simulink model "canPack_VCU_14"  (R2020a)
settings: Solver=VariableStepAuto  StartTime=0.0  StopTime=10.0  RelTol=1e-3
libraries: MyLibrary x1
settings Model: Creator=Administrator  LastModifiedBy=Administrator

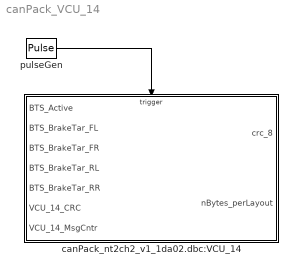
== system canPack_VCU_14 ==
  canPack_nt2ch2_v1_1da02.dbc:VCU_14 : Subsystem
  pulseGen : DiscretePulseGenerator  PulseType=Time based  Period=0.01  PulseWidth=50
  wires:
  pulseGen/1 -> canPack_nt2ch2_v1_1da02.dbc:VCU_14/Trigger

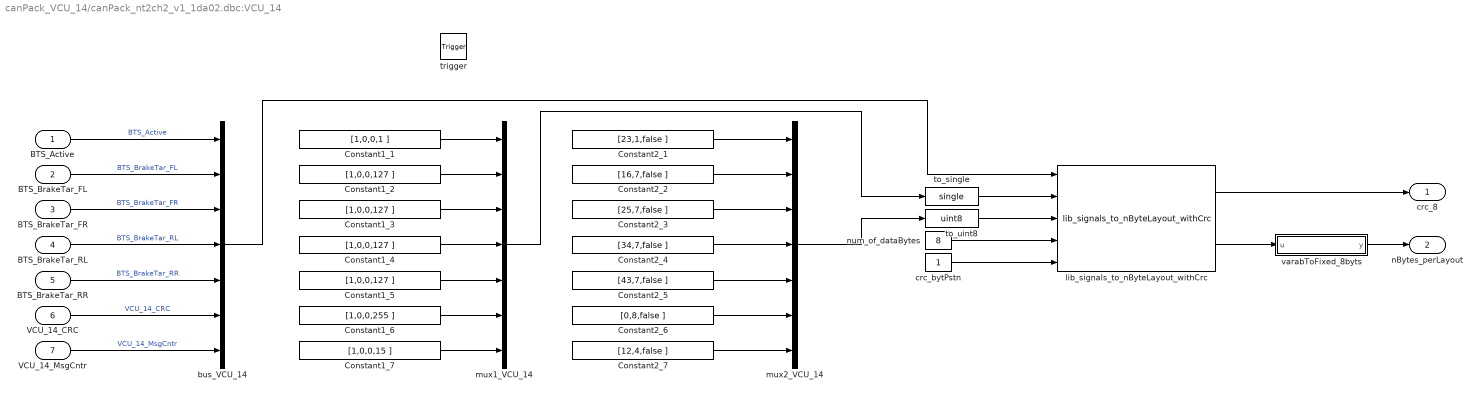
== system canPack_VCU_14/canPack_nt2ch2_v1_1da02.dbc:VCU_14 ==
  BTS_Active : Inport
  BTS_BrakeTar_FL : Inport  Port=2
  BTS_BrakeTar_FR : Inport  Port=3
  BTS_BrakeTar_RL : Inport  Port=4
  BTS_BrakeTar_RR : Inport  Port=5
  VCU_14_CRC : Inport  Port=6
  VCU_14_MsgCntr : Inport  Port=7
  trigger : TriggerPort  VariantControl=Variant  PortDimensions=1
  Constant1_1 : Constant  Value=[1,0,0,1 ]  SampleTime=-1
  Constant1_{2..5} (4 alike) : Constant  Value=[1,0,0,127 ]  SampleTime=-1
  Constant1_6 : Constant  Value=[1,0,0,255 ]  SampleTime=-1
  Constant1_7 : Constant  Value=[1,0,0,15 ]  SampleTime=-1
  Constant2_1 : Constant  Value=[23,1,false ]  SampleTime=-1
  Constant2_2 : Constant  Value=[16,7,false ]  SampleTime=-1
  Constant2_3 : Constant  Value=[25,7,false ]  SampleTime=-1
  Constant2_4 : Constant  Value=[34,7,false ]  SampleTime=-1
  Constant2_5 : Constant  Value=[43,7,false ]  SampleTime=-1
  Constant2_6 : Constant  Value=[0,8,false ]  SampleTime=-1
  Constant2_7 : Constant  Value=[12,4,false ]  SampleTime=-1
  bus_VCU_14 : BusCreator  Inputs=7
  crc_bytPstn : Constant  OutDataTypeStr=uint8  SampleTime=-1
  lib_signals_to_nByteLayout_withCrc : MyLibrary/lib_signals_to_nByteLayout_withCrc  SystemSampleTime=-1  Latency=0  AutoFrameSizeCalculation=off
  mux1_VCU_14 : Mux  Inputs=7
  mux2_VCU_14 : Mux  Inputs=7
  num_of_dataBytes : Constant  Value=8  OutDataTypeStr=uint8  SampleTime=-1
  to_single : DataTypeConversion  OutDataTypeStr=single
  to_uint8 : DataTypeConversion  OutDataTypeStr=uint8
  varabToFixed_8byts : MATLAB Function  TreatAsAtomicUnit=on
  crc_8 : Outport
  nBytes_perLayout : Outport  Port=2
  wires:
  BTS_Active/1 -> bus_VCU_14/1  "BTS_Active"
  BTS_BrakeTar_FL/1 -> bus_VCU_14/2  "BTS_BrakeTar_FL"
  BTS_BrakeTar_FR/1 -> bus_VCU_14/3  "BTS_BrakeTar_FR"
  BTS_BrakeTar_RL/1 -> bus_VCU_14/4  "BTS_BrakeTar_RL"
  BTS_BrakeTar_RR/1 -> bus_VCU_14/5  "BTS_BrakeTar_RR"
  VCU_14_CRC/1 -> bus_VCU_14/6  "VCU_14_CRC"
  VCU_14_MsgCntr/1 -> bus_VCU_14/7  "VCU_14_MsgCntr"
  Constant1_1/1 -> mux1_VCU_14/1
  Constant2_1/1 -> mux2_VCU_14/1
  Constant1_2/1 -> mux1_VCU_14/2
  Constant2_2/1 -> mux2_VCU_14/2
  Constant1_3/1 -> mux1_VCU_14/3
  Constant2_3/1 -> mux2_VCU_14/3
  Constant1_4/1 -> mux1_VCU_14/4
  Constant2_4/1 -> mux2_VCU_14/4
  Constant1_5/1 -> mux1_VCU_14/5
  Constant2_5/1 -> mux2_VCU_14/5
  Constant1_6/1 -> mux1_VCU_14/6
  Constant2_6/1 -> mux2_VCU_14/6
  Constant1_7/1 -> mux1_VCU_14/7
  Constant2_7/1 -> mux2_VCU_14/7
  bus_VCU_14/1 -> lib_signals_to_nByteLayout_withCrc/1
  mux1_VCU_14/1 -> to_single/1
  to_single/1 -> lib_signals_to_nByteLayout_withCrc/2
  mux2_VCU_14/1 -> to_uint8/1
  to_uint8/1 -> lib_signals_to_nByteLayout_withCrc/3
  lib_signals_to_nByteLayout_withCrc/1 -> crc_8/1
  num_of_dataBytes/1 -> lib_signals_to_nByteLayout_withCrc/4
  lib_signals_to_nByteLayout_withCrc/2 -> varabToFixed_8byts/1(u)
  varabToFixed_8byts/1(y) -> nBytes_perLayout/1
  crc_bytPstn/1 -> lib_signals_to_nByteLayout_withCrc/5

== matlab function canPack_VCU_14/canPack_nt2ch2_v1_1da02.dbc:VCU_14/varabToFixed_8byts ==
  data: u input uint8 size=8; y output uint8
function y = fcn(u)

fixed_size = 8;
y = uint8(zeros(fixed_size,1));

for i=1:fixed_size
    y(i) = u(i);
end
